simulink model "modelagem_cc_malha_aberta"  (R2022a)
settings: Solver=VariableStepAuto  StartTime=0.0  StopTime=10.0  RelTol=1e-3
values from neighbouring files (symbols this model uses):
  B = (Ke*Ia_vazio)/w_vazio    (= 0.00388992541754)    [determinar_tau_m.m]
  J = taum_desacelerando * B    (= 0.00162987874995)    [determinar_tau_m.m]    (also in parametros_modelo.m = 0.1)
  Ke = (Va - Ra*Ia_vazio)/w_vazio    (= 0.447346600806)    [determinar_tau_m.m]
  La = 0.001    [parametros_modelo.m]
  Ra = 3.1    [determinar_tau_m.m]    (also in parametros_modelo.m = 5.45)
settings Model: Creator=veloc  LastModifiedBy=veloc

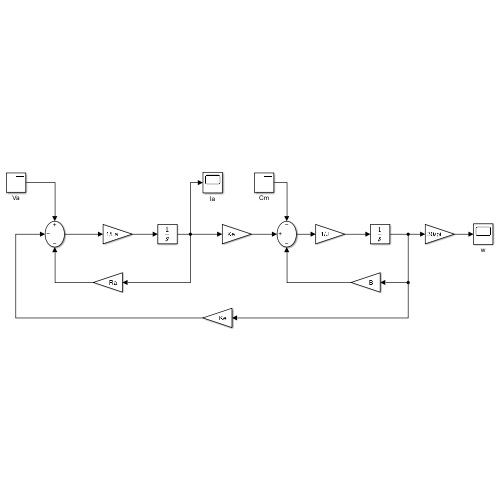
[thumbnail: Simulink's stored preview of the top-level diagram]
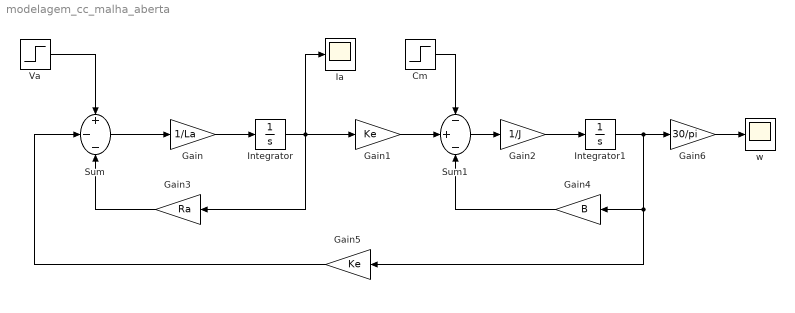
== system modelagem_cc_malha_aberta ==
  Cm : Step  Time=5  After=0.14  SampleTime=0
  Gain : Gain  Gain=1/La
  Gain1 : Gain  Gain=Ke
  Gain2 : Gain  Gain=1/J
  Gain3 : Gain  Gain=Ra
  Gain4 : Gain  Gain=B
  Gain5 : Gain  Gain=Ke
  Gain6 : Gain  Gain=30/pi
  Ia : Scope
  Integrator : Integrator
  Integrator1 : Integrator
  Sum : Sum  Inputs=+--
  Sum1 : Sum  Inputs=-+-
  Va : Step  Time=0  After=6  SampleTime=0
  w : Scope
  wires:
  Sum/1 -> Gain/1
  Gain/1 -> Integrator/1
  Integrator/1 -> Ia/1, Gain3/1, Gain1/1
  Gain2/1 -> Integrator1/1
  Integrator1/1 -> Gain5/1, Gain4/1, Gain6/1
  Va/1 -> Sum/1
  Gain1/1 -> Sum1/2
  Sum1/1 -> Gain2/1
  Cm/1 -> Sum1/1
  Gain4/1 -> Sum1/3
  Gain3/1 -> Sum/3
  Gain5/1 -> Sum/2
  Gain6/1 -> w/1
